simulink model "liftsubsystem"  (R2025b)
settings: Solver=daessc  StartTime=0.0  StopTime=15  FixedStep=1e-3  RelTol=1e-3
values from neighbouring files (symbols this model uses):
  b0 = 1.0    (= 1)    [get_arm_model_with_disturbance.m]    (also in robotParams.m = 3.125)
  beta1 = 3 * omega_o    (= 120)    [robotParams.m]
  beta2 = 3 * omega_o^2    (= 4800)    [robotParams.m]
  beta3 = omega_o^3    (= 64000)    [robotParams.m]
  g = 9.81    [get_arm_model.m]    (also in robotParams.m)
  g_fork = 2*pi*50    (= 314.159265359)    [robotParams.m]
  g_lift = 2*pi*50    (= 314.159265359)    [robotParams.m]
  Kd_fork = 5    [robotParams.m]
  Kd_lift = 5    [robotParams.m]
  Kp_fork = 20    [robotParams.m]
  Kp_lift = 20    [robotParams.m]
  lx = 0.3    [robotParams.m]
  ly = 0.8    [robotParams.m]
  lz = 1    [robotParams.m]
  m = 1    [robotParams.m]
  M = reshape([mt1,mt2,mt3],4,4)    [mass_matrix.m]    (also in robotParams.m = 16)
  m_w = 1    [robotParams.m]
  N = 20    [ocp_arm.m]    (also in ocp_arm_disturbances.m; ocp_lift.m)
  T_control = 1e-3    (= 0.001)    [robotParams.m]
undefined symbols (not defined in the file or in its folder): dspblkCoreblockFVToolHelper, gcbh, K_fd, K_fp, M_n44, Mn_33, Mn_44, X, Y, Z
libraries: sm_lib x257, nesl_utility x58, sharedTrackingLibrary x6, slpidlib x4, simulink x4, robotcorelib x1
(part 1 of 8)
settings Model: Creator=itsan  LastModifiedBy=itsan

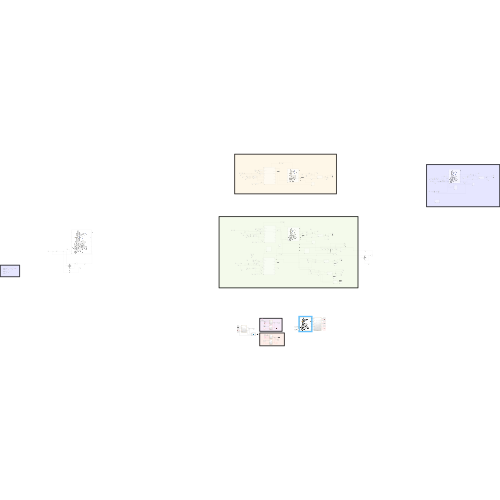
[thumbnail: Simulink's stored preview of the top-level diagram]
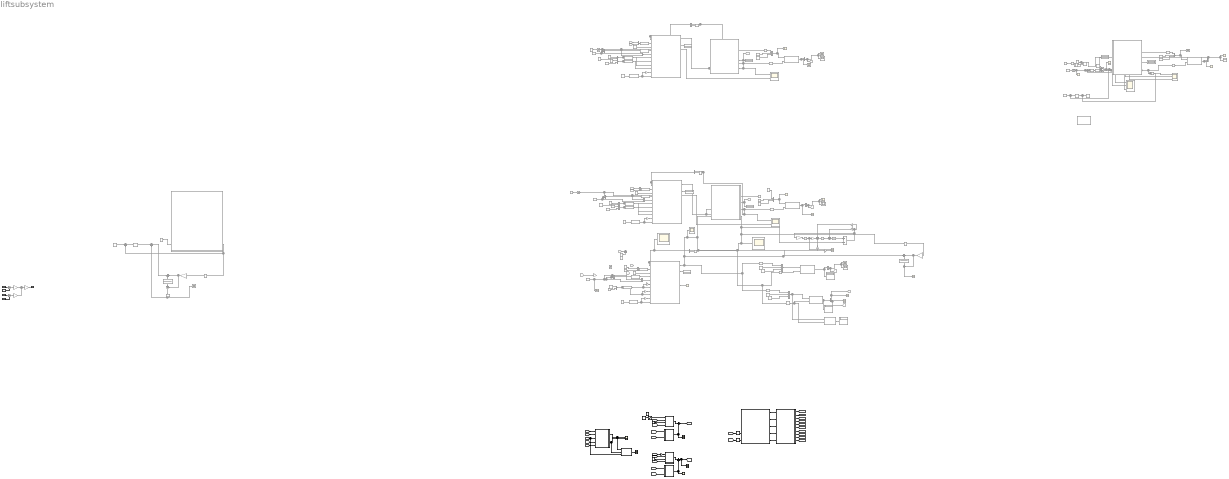
== system liftsubsystem ==
  note: Lift
  Position : Inport
  Velocity : Inport  Port=2
  Position_cmd : Inport  Port=3
  Velocity_cmd : Inport  Port=4
  Calculations : Subsystem
  Constant{,11,16,24..25} (5 alike) : Constant  Commented=on  Value=0.5
  Constant1 : Constant  Commented=on  Value=9.81
  Constant{4,10,15,26,34..35} (6 alike) : Constant  Commented=on  Value=0.01
  Constant12 : Constant  Commented=on  Value=0.8
  Constant{8,13,18,22,30,38} (6 alike) : Constant  Commented=on  Value=0
  Constant14 : Constant  Commented=on  Value=150
  Constant17 : Constant  Commented=on  Value=0.8
  Constant19 : Constant  Commented=on  Value=150
  Constant2 : Constant  Commented=on  Value=12
  Constant20 : Constant  Commented=on  Value=[0 0 0]
  Constant21 : Constant  Commented=on  Value=-0.5
  Constant{3,5,9,23} (4 alike) : Constant  Commented=on  Value=0.43
  Constant27 : Constant  Commented=on  Value=100
  Constant28 : Constant  Commented=on  Value=[0 0 0]
  Constant29 : Constant  Commented=on  Value=7
  Constant31 : Constant  Commented=on  Value=0.4
  Constant{32..33,36..37} (4 alike) : Constant  Commented=on  Value=5
  Constant39 : Constant  Commented=on  Value=-5.99
  Constant42 : Constant  Value=0
  Constant43 : Constant  Value=0
  Constant45 : Constant  Value=0.0
  Constant6 : Constant  Commented=on  Value=[0 0 0]
  Constant7 : Constant  Commented=on  Value=-0.5
  Cos : Trigonometry  Commented=on  Operator=cos
  Delay : Delay  Commented=on
  Demux{,1..3} (4 alike) : Demux  Commented=on  Outputs=3
  Demux4 : Demux  Commented=on
  Derivative{,1..5} (6 alike) : Derivative  Commented=on
  Discrete LPF1 : DiscreteFilter  Commented=on  LoadFcn=dspblkCoreblockFVToolHelper(gcbh,'load');  Numerator=[-5.866*0.001]  Denominator=[1-5.866*0.001 -1]
      settings: CopyFcn=dspblkCoreblockFVToolHelper(gcbh,'copy');  DeleteFcn=dspblkCoreblockFVToolHelper(gcbh,'close');  ModelCloseFcn=dspblkCoreblockFVToolHelper(gcbh,'close');  PreSaveFcn=dspblkCoreblockFVToolHelper(gcbh,'presave');  PostSaveFcn=dspblkCoreblockFVToolHelper(gcbh,'postsave');  CloseFcn=dspblkCoreblockFVToolHelper(gcbh,'close');
  Discrete LPF2 : DiscreteFilter  Commented=on  LoadFcn=dspblkCoreblockFVToolHelper(gcbh,'load');  Numerator=[31*0.001]  Denominator=[1+31*0.001 -1]
      settings: CopyFcn=dspblkCoreblockFVToolHelper(gcbh,'copy');  DeleteFcn=dspblkCoreblockFVToolHelper(gcbh,'close');  ModelCloseFcn=dspblkCoreblockFVToolHelper(gcbh,'close');  PreSaveFcn=dspblkCoreblockFVToolHelper(gcbh,'presave');  PostSaveFcn=dspblkCoreblockFVToolHelper(gcbh,'postsave');  CloseFcn=dspblkCoreblockFVToolHelper(gcbh,'close');
  Display{,1..13} (14 alike) : Display  Commented=on
  Divide : Product  Commented=on  Inputs=***
  Divide1 : Product  Commented=on  Inputs=**
  Extended Kalman Filter : sharedTrackingLibrary/Extended Kalman Filter  Commented=on  StateTransitionFcn=myStateTransitionFcn  HasStateTransitionJacobianFcn=off  HasAdditiveProcessNoise=Additive  ProcessNoise=diag([1e-6, 1e-4, 1e-8])  HasTimeVaryingProcessNoise=off  HasStateTransitionFcnExtraArgument=1  InitialState=[0; 0; 10]  InitialStateCovariance=diag([1e-2, 1e-2, 100])  MeasurementFcn1=myMeasurementFcn  HasMeasurementJacobianFcn1=off  HasMeasurementEnablePort1=off  HasAdditiveMeasurementNoise1=Additive  MeasurementNoise1=diag([1e-2])  HasTimeVaryingMeasurementNoise1=off  HasMeasurementFcnExtraArgument1=0  HasMeasurementWrapping1=off  MeasurementFcn2=myMeasurementFcn  HasMeasurementJacobianFcn2=off  HasMeasurementEnablePort2=off  HasAdditiveMeasurementNoise2=Additive  MeasurementNoise2=1  HasTimeVaryingMeasurementNoise2=off  HasMeasurementFcnExtraArgument2=0  HasMeasurementWrapping2=off  MeasurementFcn3=myMeasurementFcn  HasMeasurementJacobianFcn3=off  HasMeasurementEnablePort3=off  HasAdditiveMeasurementNoise3=Additive  MeasurementNoise3=1  HasTimeVaryingMeasurementNoise3=off  HasMeasurementFcnExtraArgument3=0  HasMeasurementWrapping3=off  MeasurementFcn4=myMeasurementFcn  HasMeasurementJacobianFcn4=off  HasMeasurementEnablePort4=off  HasAdditiveMeasurementNoise4=Additive  MeasurementNoise4=1  HasTimeVaryingMeasurementNoise4=off  HasMeasurementFcnExtraArgument4=0  HasMeasurementWrapping4=off  MeasurementFcn5=myMeasurementFcn  HasMeasurementJacobianFcn5=off  HasMeasurementEnablePort5=off  HasAdditiveMeasurementNoise5=Additive  MeasurementNoise5=1  HasTimeVaryingMeasurementNoise5=off  HasMeasurementFcnExtraArgument5=0  HasMeasurementWrapping5=off  EnableMultirate=off  StateTransitionFcnSampleTime=1  MeasurementFcn1SampleTime=1  MeasurementFcn2SampleTime=1  MeasurementFcn3SampleTime=1  MeasurementFcn4SampleTime=1  MeasurementFcn5SampleTime=1  UseCurrentEstimator=on  OutputStateCovariance=off  DataType=double  SampleTime=0.01  NumberOfMeasurements=1
  Extended Kalman Filter1 : sharedTrackingLibrary/Extended Kalman Filter  Commented=on  StateTransitionFcn=myStateTransitionFcn  HasStateTransitionJacobianFcn=off  HasAdditiveProcessNoise=Additive  ProcessNoise=diag([1e-6, 1e-4, 1e-8])  HasTimeVaryingProcessNoise=off  HasStateTransitionFcnExtraArgument=1  InitialState=[0; 0; 10]  InitialStateCovariance=diag([1e-2, 1e-2, 100])  MeasurementFcn1=myMeasurementFcn  HasMeasurementJacobianFcn1=off  HasMeasurementEnablePort1=off  HasAdditiveMeasurementNoise1=Additive  MeasurementNoise1=diag([1e-2])  HasTimeVaryingMeasurementNoise1=off  HasMeasurementFcnExtraArgument1=0  HasMeasurementWrapping1=off  MeasurementFcn2=myMeasurementFcn  HasMeasurementJacobianFcn2=off  HasMeasurementEnablePort2=off  HasAdditiveMeasurementNoise2=Additive  MeasurementNoise2=1  HasTimeVaryingMeasurementNoise2=off  HasMeasurementFcnExtraArgument2=0  HasMeasurementWrapping2=off  MeasurementFcn3=myMeasurementFcn  HasMeasurementJacobianFcn3=off  HasMeasurementEnablePort3=off  HasAdditiveMeasurementNoise3=Additive  MeasurementNoise3=1  HasTimeVaryingMeasurementNoise3=off  HasMeasurementFcnExtraArgument3=0  HasMeasurementWrapping3=off  MeasurementFcn4=myMeasurementFcn  HasMeasurementJacobianFcn4=off  HasMeasurementEnablePort4=off  HasAdditiveMeasurementNoise4=Additive  MeasurementNoise4=1  HasTimeVaryingMeasurementNoise4=off  HasMeasurementFcnExtraArgument4=0  HasMeasurementWrapping4=off  MeasurementFcn5=myMeasurementFcn  HasMeasurementJacobianFcn5=off  HasMeasurementEnablePort5=off  HasAdditiveMeasurementNoise5=Additive  MeasurementNoise5=1  HasTimeVaryingMeasurementNoise5=off  HasMeasurementFcnExtraArgument5=0  HasMeasurementWrapping5=off  EnableMultirate=off  StateTransitionFcnSampleTime=1  MeasurementFcn1SampleTime=1  MeasurementFcn2SampleTime=1  MeasurementFcn3SampleTime=1  MeasurementFcn4SampleTime=1  MeasurementFcn5SampleTime=1  UseCurrentEstimator=on  OutputStateCovariance=off  DataType=double  SampleTime=0.01  NumberOfMeasurements=1
  Extended Kalman Filter2 : sharedTrackingLibrary/Extended Kalman Filter  Commented=on  StateTransitionFcn=liftStateTransitionFcn  HasStateTransitionJacobianFcn=off  HasAdditiveProcessNoise=Additive  ProcessNoise=diag([1e-6, 1e-4, 1e-8])  HasTimeVaryingProcessNoise=off  HasStateTransitionFcnExtraArgument=1  InitialState=[0; 0; 10]  InitialStateCovariance=diag([1e-2, 1e-2, 100])  MeasurementFcn1=liftMeasurementFcn  HasMeasurementJacobianFcn1=off  HasMeasurementEnablePort1=off  HasAdditiveMeasurementNoise1=Additive  MeasurementNoise1=diag([1e-2])  HasTimeVaryingMeasurementNoise1=off  HasMeasurementFcnExtraArgument1=0  HasMeasurementWrapping1=off  MeasurementFcn2=myMeasurementFcn  HasMeasurementJacobianFcn2=off  HasMeasurementEnablePort2=off  HasAdditiveMeasurementNoise2=Additive  MeasurementNoise2=1  HasTimeVaryingMeasurementNoise2=off  HasMeasurementFcnExtraArgument2=0  HasMeasurementWrapping2=off  MeasurementFcn3=myMeasurementFcn  HasMeasurementJacobianFcn3=off  HasMeasurementEnablePort3=off  HasAdditiveMeasurementNoise3=Additive  MeasurementNoise3=1  HasTimeVaryingMeasurementNoise3=off  HasMeasurementFcnExtraArgument3=0  HasMeasurementWrapping3=off  MeasurementFcn4=myMeasurementFcn  HasMeasurementJacobianFcn4=off  HasMeasurementEnablePort4=off  HasAdditiveMeasurementNoise4=Additive  MeasurementNoise4=1  HasTimeVaryingMeasurementNoise4=off  HasMeasurementFcnExtraArgument4=0  HasMeasurementWrapping4=off  MeasurementFcn5=myMeasurementFcn  HasMeasurementJacobianFcn5=off  HasMeasurementEnablePort5=off  HasAdditiveMeasurementNoise5=Additive  MeasurementNoise5=1  HasTimeVaryingMeasurementNoise5=off  HasMeasurementFcnExtraArgument5=0  HasMeasurementWrapping5=off  EnableMultirate=off  StateTransitionFcnSampleTime=1  MeasurementFcn1SampleTime=1  MeasurementFcn2SampleTime=1  MeasurementFcn3SampleTime=1  MeasurementFcn4SampleTime=1  MeasurementFcn5SampleTime=1  UseCurrentEstimator=on  OutputStateCovariance=off  DataType=double  SampleTime=0.01  NumberOfMeasurements=1
  Extended Kalman Filter3 : sharedTrackingLibrary/Extended Kalman Filter  Commented=on  StateTransitionFcn=armStateTransitionFcn  HasStateTransitionJacobianFcn=off  HasAdditiveProcessNoise=Additive  ProcessNoise=diag([1e-8, 1e-6,1e-10])  HasTimeVaryingProcessNoise=off  HasStateTransitionFcnExtraArgument=1  InitialState=[0;0;0.3]  InitialStateCovariance=diag([1e-4, 1e-4,100])  MeasurementFcn1=armMeasurementFcn  HasMeasurementJacobianFcn1=off  HasMeasurementEnablePort1=off  HasAdditiveMeasurementNoise1=Additive  MeasurementNoise1=1e-4  HasTimeVaryingMeasurementNoise1=off  HasMeasurementFcnExtraArgument1=0  HasMeasurementWrapping1=off  MeasurementFcn2=myMeasurementFcn  HasMeasurementJacobianFcn2=off  HasMeasurementEnablePort2=off  HasAdditiveMeasurementNoise2=Additive  MeasurementNoise2=1  HasTimeVaryingMeasurementNoise2=off  HasMeasurementFcnExtraArgument2=0  HasMeasurementWrapping2=off  MeasurementFcn3=myMeasurementFcn  HasMeasurementJacobianFcn3=off  HasMeasurementEnablePort3=off  HasAdditiveMeasurementNoise3=Additive  MeasurementNoise3=1  HasTimeVaryingMeasurementNoise3=off  HasMeasurementFcnExtraArgument3=0  HasMeasurementWrapping3=off  MeasurementFcn4=myMeasurementFcn  HasMeasurementJacobianFcn4=off  HasMeasurementEnablePort4=off  HasAdditiveMeasurementNoise4=Additive  MeasurementNoise4=1  HasTimeVaryingMeasurementNoise4=off  HasMeasurementFcnExtraArgument4=0  HasMeasurementWrapping4=off  MeasurementFcn5=myMeasurementFcn  HasMeasurementJacobianFcn5=off  HasMeasurementEnablePort5=off  HasAdditiveMeasurementNoise5=Additive  MeasurementNoise5=1  HasTimeVaryingMeasurementNoise5=off  HasMeasurementFcnExtraArgument5=0  HasMeasurementWrapping5=off  EnableMultirate=off  StateTransitionFcnSampleTime=1  MeasurementFcn1SampleTime=1  MeasurementFcn2SampleTime=1  MeasurementFcn3SampleTime=1  MeasurementFcn4SampleTime=1  MeasurementFcn5SampleTime=1  UseCurrentEstimator=on  OutputStateCovariance=off  DataType=double  SampleTime=0.01  NumberOfMeasurements=1
  Extended Kalman Filter5 : sharedTrackingLibrary/Extended Kalman Filter  Commented=on  StateTransitionFcn=armMassStateTransitionFcn  HasStateTransitionJacobianFcn=off  HasAdditiveProcessNoise=Additive  ProcessNoise=diag([1e-8, 1e-6,1e-10,1e-10])  HasTimeVaryingProcessNoise=off  HasStateTransitionFcnExtraArgument=1  InitialState=[0;0;0.3;2]  InitialStateCovariance=diag([1e-4, 1e-4,100,100])  MeasurementFcn1=armMeasurementFcn  HasMeasurementJacobianFcn1=off  HasMeasurementEnablePort1=off  HasAdditiveMeasurementNoise1=Additive  MeasurementNoise1=1e-4  HasTimeVaryingMeasurementNoise1=off  HasMeasurementFcnExtraArgument1=0  HasMeasurementWrapping1=off  MeasurementFcn2=myMeasurementFcn  HasMeasurementJacobianFcn2=off  HasMeasurementEnablePort2=off  HasAdditiveMeasurementNoise2=Additive  MeasurementNoise2=1  HasTimeVaryingMeasurementNoise2=off  HasMeasurementFcnExtraArgument2=0  HasMeasurementWrapping2=off  MeasurementFcn3=myMeasurementFcn  HasMeasurementJacobianFcn3=off  HasMeasurementEnablePort3=off  HasAdditiveMeasurementNoise3=Additive  MeasurementNoise3=1  HasTimeVaryingMeasurementNoise3=off  HasMeasurementFcnExtraArgument3=0  HasMeasurementWrapping3=off  MeasurementFcn4=myMeasurementFcn  HasMeasurementJacobianFcn4=off  HasMeasurementEnablePort4=off  HasAdditiveMeasurementNoise4=Additive  MeasurementNoise4=1  HasTimeVaryingMeasurementNoise4=off  HasMeasurementFcnExtraArgument4=0  HasMeasurementWrapping4=off  MeasurementFcn5=myMeasurementFcn  HasMeasurementJacobianFcn5=off  HasMeasurementEnablePort5=off  HasAdditiveMeasurementNoise5=Additive  MeasurementNoise5=1  HasTimeVaryingMeasurementNoise5=off  HasMeasurementFcnExtraArgument5=0  HasMeasurementWrapping5=off  EnableMultirate=off  StateTransitionFcnSampleTime=1  MeasurementFcn1SampleTime=1  MeasurementFcn2SampleTime=1  MeasurementFcn3SampleTime=1  MeasurementFcn4SampleTime=1  MeasurementFcn5SampleTime=1  UseCurrentEstimator=on  OutputStateCovariance=off  DataType=double  SampleTime=0.01  NumberOfMeasurements=1
  Fork DOB : Subsystem
  From{,2,6..7} (4 alike) : From  Commented=on  GotoTag=Mass
  From1 : From  Commented=on  GotoTag=Pitch
  From3 : From  Commented=on  GotoTag=Pitch
  From4 : From  Commented=on  GotoTag=Pitch
  From5 : From  Commented=on  GotoTag=rx
  Gain{,1..5,12} (7 alike) : Gain  Commented=on  Gain=-1
  Gain10 : Gain  Commented=on  Gain=b0
  Gain11 : Gain  Commented=on  Gain=beta2
  Gain13 : Gain  Commented=on  Gain=beta1
  Gain14 : Gain  Commented=on  Gain=-beta3
  Gain15 : Gain  Commented=on  Gain=b0
  Gain16 : Gain  Commented=on  Gain=31*0.21
  Gain18 : Gain  Gain=-1
  Gain6 : Gain  Commented=on  Gain=K_fp
  Gain7 : Gain  Commented=on  Gain=K_fd
  Gain8 : Gain  Commented=on  Gain=M_n44
  Gain9 : Gain  Commented=on  Gain=-0.21*5.866
  Goto : Goto  Commented=on  GotoTag=Mass
  Goto1 : Goto  Commented=on  GotoTag=Pitch
  Goto2 : Goto  Commented=on  GotoTag=Mass
  Goto3 : Goto  Commented=on  GotoTag=Pitch
  Goto4 : Goto  Commented=on  GotoTag=Mass
  Goto5 : Goto  Commented=on  GotoTag=rx
  Goto6 : Goto  Commented=on  GotoTag=rx
  Lift DOB : Subsystem
  MATLAB Function : MATLAB Function  TreatAsAtomicUnit=on
  Mux{,2,5..8,10,12..15,18..20} (14 alike) : Mux  Commented=on  Inputs=2
  Mux{1,3..4,9,11,16..17,21} (8 alike) : Mux  Commented=on  Inputs=3
  PD : slpidlib/PID Controller  Commented=on  Controller=PID  Form=Parallel  TimeDomain=Continuous-time  UseExternalTs=off  SampleTime=-1  IntegratorMethod=Forward Euler  FilterMethod=Forward Euler  ControllerParametersSource=internal  P=1  I=0.001  UseKiTs=off  D=22  UseExternalDerivativeSource=off  N=15  UseFilter=on  TunerSelectOption=Transfer Function Based (PID Tuner App)  InitialConditionSource=internal  InitialConditionForIntegrator=0  InitialConditionForFilter=0  DifferentiatorICPrevScaledInput=0  ExternalReset=none  TrackingMode=off  Kt=1  LimitOutput=on  SatLimitsSource=internal  UpperSaturationLimit=100  LowerSaturationLimit=-100  LinearizeAsGain=on  AntiWindupMode=back-calculation  Kb=3  LimitIntegrator=off  UpperIntegratorSaturationLimit=inf  LowerIntegratorSaturationLimit=-inf  POutMin=[]  POutMax=[]  IOutMin=[]  IOutMax=[]  DOutMin=[]  DOutMax=[]  NOutMin=[]  NOutMax=[]  SumOutMin=[]  SumOutMax=[]  SaturationOutMin=[]  SaturationOutMax=[]  PParamMin=[]  PParamMax=[]  IParamMin=[]  IParamMax=[]  DParamMin=[]  DParamMax=[]  NParamMin=[]  NParamMax=[]  KbParamMin=[]  KbParamMax=[]  KtParamMin=[]  KtParamMax=[]  KbOutMin=[]  KbOutMax=[]  KtOutMin=[]  KtOutMax=[]  IntegratorOutMin=[]  IntegratorOutMax=[]  FilterOutMin=[]  FilterOutMax=[]  SumI1OutMin=[]  SumI1OutMax=[]  SumI2OutMin=[]  SumI2OutMax=[]  SumI3OutMin=[]  SumI3OutMax=[]  SumI4OutMin=[]  SumI4OutMax=[]  SumDOutMin=[]  SumDOutMax=[]  DifferentiatorOutMin=[]  DifferentiatorOutMax=[]  FilterDiffOutCoefMin=[]  FilterDiffOutCoefMax=[]  ReciprocalOutMin=[]  ReciprocalOutMax=[]  SumDenOutMin=[]  SumDenOutMax=[]  SumNumOutMin=[]  SumNumOutMax=[]  DivideOutMin=[]  DivideOutMax=[]  UdiffTsProdOutMin=[]  UdiffTsProdOutMax=[]  NTsProdOutMin=[]  NTsProdOutMax=[]  UintegralTsProdOutMin=[]  UintegralTsProdOutMax=[]  UngainTsProdOutMin=[]  UngainTsProdOutMax=[]  ClampingZeroOutDataTypeStr=Inherit: Inherit via back propagation  ClampingZeroOutMin=[]  ClampingZeroOutMax=[]  FilterDenConstantOutDataTypeStr=Inherit: Inherit via back propagation  FilterDenConstantOutMin=[]  FilterDenConstantOutMax=[]  PCopyOutDataTypeStr=Inherit: Inherit via back propagation  PCopyOutMin=[]  PCopyOutMax=[]  NCopyOutDataTypeStr=Inherit: Inherit via back propagation  NCopyOutMin=[]  NCopyOutMax=[]  IntegratorContinuousStateAttributes=''  IntegratorStateMustResolveToSignalObject=off  IntegratorRTWStateStorageClass=Auto  FilterContinuousStateAttributes=''  FilterStateMustResolveToSignalObject=off  FilterRTWStateStorageClass=Auto  ParallelPVariant=InternalParameters  IdealPVariant=Disabled  IVariant=InternalParameters  DVariant=InternalParameters  IntegratorVariant=Continuous  SatVariant=Enabled  AWVariant=BackCalculation  PCopyVariant=Disabled  TRVariant=Disabled  FdbkBlocksVariant=Forward  IdealPFdbkVariant=Disabled  SatFdbkVariant=Disabled  DerivativeFilterVariant=ContFilter  NVariant=InternalParameters  NCopyVariant=Disabled  FilterICVariant=InternalICsFilter  IntegratorICVariant=InternalICs  ExternalResetVariant=Disabled  TRSumVariant=Passthrough  SumFdbkVariant=Disabled  SumVariant=Sum_PID  TsampFilterVariant=InternalTs  TsampNgainVariant=Passthrough  TsampIntegralVariant=Disabled_SignalSpec  ExternalSaturationOutDataTypeStr=Inherit: Same as second input  DerivativeSourceVariant=ErrorSignal  PreIntVariant=InternalPreInt
  PD fork : Subsystem
  PD lift : Subsystem
  PID Controller : slpidlib/PID Controller  Commented=on  Controller=PID  Form=Parallel  TimeDomain=Continuous-time  UseExternalTs=off  SampleTime=-1  IntegratorMethod=Forward Euler  FilterMethod=Forward Euler  ControllerParametersSource=internal  P=10  I=0  UseKiTs=off  D=0  UseExternalDerivativeSource=off  N=0  UseFilter=on  TunerSelectOption=Transfer Function Based (PID Tuner App)  InitialConditionSource=internal  InitialConditionForIntegrator=0  InitialConditionForFilter=0  DifferentiatorICPrevScaledInput=0  ExternalReset=none  TrackingMode=off  Kt=1  LimitOutput=on  SatLimitsSource=internal  UpperSaturationLimit=1  LowerSaturationLimit=-1  LinearizeAsGain=on  AntiWindupMode=none  Kb=1  LimitIntegrator=off  UpperIntegratorSaturationLimit=inf  LowerIntegratorSaturationLimit=-inf  POutMin=[]  POutMax=[]  IOutMin=[]  IOutMax=[]  DOutMin=[]  DOutMax=[]  NOutMin=[]  NOutMax=[]  SumOutMin=[]  SumOutMax=[]  SaturationOutMin=[]  SaturationOutMax=[]  PParamMin=[]  PParamMax=[]  IParamMin=[]  IParamMax=[]  DParamMin=[]  DParamMax=[]  NParamMin=[]  NParamMax=[]  KbParamMin=[]  KbParamMax=[]  KtParamMin=[]  KtParamMax=[]  KbOutMin=[]  KbOutMax=[]  KtOutMin=[]  KtOutMax=[]  IntegratorOutMin=[]  IntegratorOutMax=[]  FilterOutMin=[]  FilterOutMax=[]  SumI1OutMin=[]  SumI1OutMax=[]  SumI2OutMin=[]  SumI2OutMax=[]  SumI3OutMin=[]  SumI3OutMax=[]  SumI4OutMin=[]  SumI4OutMax=[]  SumDOutMin=[]  SumDOutMax=[]  DifferentiatorOutMin=[]  DifferentiatorOutMax=[]  FilterDiffOutCoefMin=[]  FilterDiffOutCoefMax=[]  ReciprocalOutMin=[]  ReciprocalOutMax=[]  SumDenOutMin=[]  SumDenOutMax=[]  SumNumOutMin=[]  SumNumOutMax=[]  DivideOutMin=[]  DivideOutMax=[]  UdiffTsProdOutMin=[]  UdiffTsProdOutMax=[]  NTsProdOutMin=[]  NTsProdOutMax=[]  UintegralTsProdOutMin=[]  UintegralTsProdOutMax=[]  UngainTsProdOutMin=[]  UngainTsProdOutMax=[]  ClampingZeroOutDataTypeStr=Inherit: Inherit via back propagation  ClampingZeroOutMin=[]  ClampingZeroOutMax=[]  FilterDenConstantOutDataTypeStr=Inherit: Inherit via back propagation  FilterDenConstantOutMin=[]  FilterDenConstantOutMax=[]  PCopyOutDataTypeStr=Inherit: Inherit via back propagation  PCopyOutMin=[]  PCopyOutMax=[]  NCopyOutDataTypeStr=Inherit: Inherit via back propagation  NCopyOutMin=[]  NCopyOutMax=[]  IntegratorContinuousStateAttributes=''  IntegratorStateMustResolveToSignalObject=off  IntegratorRTWStateStorageClass=Auto  FilterContinuousStateAttributes=''  FilterStateMustResolveToSignalObject=off  FilterRTWStateStorageClass=Auto  ParallelPVariant=InternalParameters  IdealPVariant=Disabled  IVariant=InternalParameters  DVariant=InternalParameters  IntegratorVariant=Continuous  SatVariant=Enabled  AWVariant=Passthrough  PCopyVariant=Disabled  TRVariant=Disabled  FdbkBlocksVariant=Forward  IdealPFdbkVariant=Disabled  SatFdbkVariant=Disabled  DerivativeFilterVariant=ContFilter  NVariant=InternalParameters  NCopyVariant=Disabled  FilterICVariant=InternalICsFilter  IntegratorICVariant=InternalICs  ExternalResetVariant=Disabled  TRSumVariant=Passthrough  SumFdbkVariant=Disabled  SumVariant=Sum_PID  TsampFilterVariant=InternalTs  TsampNgainVariant=Passthrough  TsampIntegralVariant=Disabled_SignalSpec  ExternalSaturationOutDataTypeStr=Inherit: Same as second input  DerivativeSourceVariant=ErrorSignal  PreIntVariant=InternalPreInt
  PID Controller1 : slpidlib/PID Controller  Commented=on  Controller=PID  Form=Parallel  TimeDomain=Continuous-time  UseExternalTs=off  SampleTime=-1  IntegratorMethod=Forward Euler  FilterMethod=Forward Euler  ControllerParametersSource=internal  P=10  I=4  UseKiTs=off  D=0  UseExternalDerivativeSource=off  N=0  UseFilter=on  TunerSelectOption=Transfer Function Based (PID Tuner App)  InitialConditionSource=internal  InitialConditionForIntegrator=0  InitialConditionForFilter=0  DifferentiatorICPrevScaledInput=0  ExternalReset=none  TrackingMode=off  Kt=1  LimitOutput=on  SatLimitsSource=internal  UpperSaturationLimit=1  LowerSaturationLimit=-1  LinearizeAsGain=on  AntiWindupMode=none  Kb=1  LimitIntegrator=off  UpperIntegratorSaturationLimit=inf  LowerIntegratorSaturationLimit=-inf  POutMin=[]  POutMax=[]  IOutMin=[]  IOutMax=[]  DOutMin=[]  DOutMax=[]  NOutMin=[]  NOutMax=[]  SumOutMin=[]  SumOutMax=[]  SaturationOutMin=[]  SaturationOutMax=[]  PParamMin=[]  PParamMax=[]  IParamMin=[]  IParamMax=[]  DParamMin=[]  DParamMax=[]  NParamMin=[]  NParamMax=[]  KbParamMin=[]  KbParamMax=[]  KtParamMin=[]  KtParamMax=[]  KbOutMin=[]  KbOutMax=[]  KtOutMin=[]  KtOutMax=[]  IntegratorOutMin=[]  IntegratorOutMax=[]  FilterOutMin=[]  FilterOutMax=[]  SumI1OutMin=[]  SumI1OutMax=[]  SumI2OutMin=[]  SumI2OutMax=[]  SumI3OutMin=[]  SumI3OutMax=[]  SumI4OutMin=[]  SumI4OutMax=[]  SumDOutMin=[]  SumDOutMax=[]  DifferentiatorOutMin=[]  DifferentiatorOutMax=[]  FilterDiffOutCoefMin=[]  FilterDiffOutCoefMax=[]  ReciprocalOutMin=[]  ReciprocalOutMax=[]  SumDenOutMin=[]  SumDenOutMax=[]  SumNumOutMin=[]  SumNumOutMax=[]  DivideOutMin=[]  DivideOutMax=[]  UdiffTsProdOutMin=[]  UdiffTsProdOutMax=[]  NTsProdOutMin=[]  NTsProdOutMax=[]  UintegralTsProdOutMin=[]  UintegralTsProdOutMax=[]  UngainTsProdOutMin=[]  UngainTsProdOutMax=[]  ClampingZeroOutDataTypeStr=Inherit: Inherit via back propagation  ClampingZeroOutMin=[]  ClampingZeroOutMax=[]  FilterDenConstantOutDataTypeStr=Inherit: Inherit via back propagation  FilterDenConstantOutMin=[]  FilterDenConstantOutMax=[]  PCopyOutDataTypeStr=Inherit: Inherit via back propagation  PCopyOutMin=[]  PCopyOutMax=[]  NCopyOutDataTypeStr=Inherit: Inherit via back propagation  NCopyOutMin=[]  NCopyOutMax=[]  IntegratorContinuousStateAttributes=''  IntegratorStateMustResolveToSignalObject=off  IntegratorRTWStateStorageClass=Auto  FilterContinuousStateAttributes=''  FilterStateMustResolveToSignalObject=off  FilterRTWStateStorageClass=Auto  ParallelPVariant=InternalParameters  IdealPVariant=Disabled  IVariant=InternalParameters  DVariant=InternalParameters  IntegratorVariant=Continuous  SatVariant=Enabled  AWVariant=Passthrough  PCopyVariant=Disabled  TRVariant=Disabled  FdbkBlocksVariant=Forward  IdealPFdbkVariant=Disabled  SatFdbkVariant=Disabled  DerivativeFilterVariant=ContFilter  NVariant=InternalParameters  NCopyVariant=Disabled  FilterICVariant=InternalICsFilter  IntegratorICVariant=InternalICs  ExternalResetVariant=Disabled  TRSumVariant=Passthrough  SumFdbkVariant=Disabled  SumVariant=Sum_PID  TsampFilterVariant=InternalTs  TsampNgainVariant=Passthrough  TsampIntegralVariant=Disabled_SignalSpec  ExternalSaturationOutDataTypeStr=Inherit: Same as second input  DerivativeSourceVariant=ErrorSignal  PreIntVariant=InternalPreInt
  PID Controller2 : slpidlib/PID Controller  Commented=on  Controller=PID  Form=Parallel  TimeDomain=Continuous-time  UseExternalTs=off  SampleTime=-1  IntegratorMethod=Forward Euler  FilterMethod=Forward Euler  ControllerParametersSource=internal  P=1  I=0  UseKiTs=off  D=1  UseExternalDerivativeSource=off  N=100  UseFilter=on  TunerSelectOption=Transfer Function Based (PID Tuner App)  InitialConditionSource=internal  InitialConditionForIntegrator=0  InitialConditionForFilter=0  DifferentiatorICPrevScaledInput=0  ExternalReset=none  TrackingMode=off  Kt=1  LimitOutput=off  SatLimitsSource=internal  UpperSaturationLimit=inf  LowerSaturationLimit=-inf  LinearizeAsGain=on  AntiWindupMode=none  Kb=1  LimitIntegrator=off  UpperIntegratorSaturationLimit=inf  LowerIntegratorSaturationLimit=-inf  POutMin=[]  POutMax=[]  IOutMin=[]  IOutMax=[]  DOutMin=[]  DOutMax=[]  NOutMin=[]  NOutMax=[]  SumOutMin=[]  SumOutMax=[]  SaturationOutMin=[]  SaturationOutMax=[]  PParamMin=[]  PParamMax=[]  IParamMin=[]  IParamMax=[]  DParamMin=[]  DParamMax=[]  NParamMin=[]  NParamMax=[]  KbParamMin=[]  KbParamMax=[]  KtParamMin=[]  KtParamMax=[]  KbOutMin=[]  KbOutMax=[]  KtOutMin=[]  KtOutMax=[]  IntegratorOutMin=[]  IntegratorOutMax=[]  FilterOutMin=[]  FilterOutMax=[]  SumI1OutMin=[]  SumI1OutMax=[]  SumI2OutMin=[]  SumI2OutMax=[]  SumI3OutMin=[]  SumI3OutMax=[]  SumI4OutMin=[]  SumI4OutMax=[]  SumDOutMin=[]  SumDOutMax=[]  DifferentiatorOutMin=[]  DifferentiatorOutMax=[]  FilterDiffOutCoefMin=[]  FilterDiffOutCoefMax=[]  ReciprocalOutMin=[]  ReciprocalOutMax=[]  SumDenOutMin=[]  SumDenOutMax=[]  SumNumOutMin=[]  SumNumOutMax=[]  DivideOutMin=[]  DivideOutMax=[]  UdiffTsProdOutMin=[]  UdiffTsProdOutMax=[]  NTsProdOutMin=[]  NTsProdOutMax=[]  UintegralTsProdOutMin=[]  UintegralTsProdOutMax=[]  UngainTsProdOutMin=[]  UngainTsProdOutMax=[]  ClampingZeroOutDataTypeStr=Inherit: Inherit via back propagation  ClampingZeroOutMin=[]  ClampingZeroOutMax=[]  FilterDenConstantOutDataTypeStr=Inherit: Inherit via back propagation  FilterDenConstantOutMin=[]  FilterDenConstantOutMax=[]  PCopyOutDataTypeStr=Inherit: Inherit via back propagation  PCopyOutMin=[]  PCopyOutMax=[]  NCopyOutDataTypeStr=Inherit: Inherit via back propagation  NCopyOutMin=[]  NCopyOutMax=[]  IntegratorContinuousStateAttributes=''  IntegratorStateMustResolveToSignalObject=off  IntegratorRTWStateStorageClass=Auto  FilterContinuousStateAttributes=''  FilterStateMustResolveToSignalObject=off  FilterRTWStateStorageClass=Auto  ParallelPVariant=InternalParameters  IdealPVariant=Disabled  IVariant=InternalParameters  DVariant=InternalParameters  IntegratorVariant=Continuous  SatVariant=Disabled  AWVariant=Passthrough  PCopyVariant=Disabled  TRVariant=Disabled  FdbkBlocksVariant=Forward  IdealPFdbkVariant=Disabled  SatFdbkVariant=Disabled  DerivativeFilterVariant=ContFilter  NVariant=InternalParameters  NCopyVariant=Disabled  FilterICVariant=InternalICsFilter  IntegratorICVariant=InternalICs  ExternalResetVariant=Disabled  TRSumVariant=Passthrough  SumFdbkVariant=Disabled  SumVariant=Sum_PID  TsampFilterVariant=InternalTs  TsampNgainVariant=Passthrough  TsampIntegralVariant=Disabled_SignalSpec  ExternalSaturationOutDataTypeStr=Inherit: Same as second input  DerivativeSourceVariant=ErrorSignal  PreIntVariant=InternalPreInt
  Plant1 : Subsystem  Commented=on
      mask Display: image('plant.png');
  Plant2 : Subsystem  Commented=on
      mask Display: image('plant.png');
  Plant3 : Subsystem  Commented=on
      mask Display: image('plant.png');
  Plant4 : Subsystem  Commented=on
      mask Display: image('plant.png');
  Plant5 : Subsystem
      mask Display: image('plant.png');
  Ramp : simulink/Sources/Ramp  Commented=on  slope=0.5  start=0  InitialOutput=0
  Ramp1 : simulink/Sources/Ramp  Commented=on  slope=1  start=0  InitialOutput=0
  Ramp2 : simulink/Sources/Ramp  slope=0.05  start=1  InitialOutput=0
  Ramp3 : simulink/Sources/Ramp  Commented=on  slope=1  start=0  InitialOutput=0
  Rate Transition : RateTransition  OutPortSampleTime=T_control
  Rate Transition1 : RateTransition  OutPortSampleTime=T_control
  S-Function : S-Function  Commented=on  FunctionName=repmat_sfun  Parameters=N+1  SFunctionDeploymentMode=off  EnableBusSupport=off
  S-Function1 : S-Function  Commented=on  FunctionName=acados_solver_sfunction_linear_actuator_model  SFunctionDeploymentMode=off  EnableBusSupport=off
      mask Display:
      | % from the make_sfun file
      | global sfun_input_names sfun_output_names
      | for i = 1:length(sfun_input_names)
      | 	port_label('input', i, sfun_input_names{i})
      | end
      | for i = 1:length(sfun_output_names)
      | 	port_label('output', i, sfun_output_names{i})
      | end
  S-Function{2..4,8..10,12,16} (8 alike) : S-Function  Commented=on  FunctionName=repmat_sfun  Parameters=N-1  SFunctionDeploymentMode=off  EnableBusSupport=off
  S-Function11 : S-Function  Commented=on  FunctionName=repmat_sfun  Parameters=N  SFunctionDeploymentMode=off  EnableBusSupport=off
  S-Function13 : S-Function  Commented=on  FunctionName=repmat_sfun  Parameters=N  SFunctionDeploymentMode=off  EnableBusSupport=off
  S-Function14 : S-Function  Commented=on  FunctionName=repmat_sfun  Parameters=N+1  SFunctionDeploymentMode=off  EnableBusSupport=off
  S-Function15 : S-Function  Commented=on  FunctionName=acados_solver_sfunction_arm_model  SFunctionDeploymentMode=off  EnableBusSupport=off
      mask Display:
      | % from the make_sfun file
      | global sfun_input_names sfun_output_names
      | for i = 1:length(sfun_input_names)
      | 	port_label('input', i, sfun_input_names{i})
      | end
      | for i = 1:length(sfun_output_names)
      | 	port_label('output', i, sfun_output_names{i})
      | end
  S-Function5 : S-Function  Commented=on  FunctionName=repmat_sfun  Parameters=N  SFunctionDeploymentMode=off  EnableBusSupport=off
  S-Function6 : S-Function  Commented=on  FunctionName=repmat_sfun  Parameters=N+1  SFunctionDeploymentMode=off  EnableBusSupport=off
  S-Function7 : S-Function  Commented=on  FunctionName=acados_solver_sfunction_linear_actuator_model  SFunctionDeploymentMode=off  EnableBusSupport=off
      mask Display:
      | % from the make_sfun file
      | global sfun_input_names sfun_output_names
      | for i = 1:length(sfun_input_names)
      | 	port_label('input', i, sfun_input_names{i})
      | end
      | for i = 1:length(sfun_output_names)
      | 	port_label('output', i, sfun_output_names{i})
      | end
  Saturation : Saturate  Commented=on
  Saturation1 : Saturate  Commented=on
  Saturation2 : Saturate  UpperLimit=.25
  Saturation3 : Saturate  Commented=on  UpperLimit=0.1
  Scope{,2..4,6,8..11,13..23,25} (21 alike) : Scope  Commented=on
      Scope settings: ActiveDisplayYMinimum=117.38726606594429  ActiveDisplayYMaximum=117.96497291719386
      Scope10 settings: ActiveDisplayYMinimum=10.368033685081326  ActiveDisplayYMaximum=13.754521835601309  DataLoggingVariableName=ScopeData7
      Scope11 settings: ActiveDisplayYMinimum=-23.500486572497707  ActiveDisplayYMaximum=44.300288166456191  DataLoggingVariableName=ScopeData9
      Scope13 settings: ActiveDisplayYMinimum=-23.500486572497707  ActiveDisplayYMaximum=44.300288166456191  DataLoggingVariableName=ScopeData10
      Scope14 settings: ActiveDisplayYMinimum=-23.500486572497707  ActiveDisplayYMaximum=44.300288166456191  DataLoggingVariableName=ScopeData12
      Scope15 settings: ActiveDisplayYMinimum=-1  ActiveDisplayYMaximum=1  DataLoggingVariableName=ScopeData21
      Scope16 settings: ActiveDisplayYMinimum=-0.065967569407599264  ActiveDisplayYMaximum=0.0325873905390409  DataLoggingVariableName=ScopeData22
      Scope17 settings: ActiveDisplayYMinimum=-12.264920720176846  ActiveDisplayYMaximum=-8.5595612380933073  DataLoggingVariableName=ScopeData23
      Scope18 settings: ActiveDisplayYMinimum=-0.06438015181759206  ActiveDisplayYMaximum=0.57942136635832864  DataLoggingVariableName=ScopeData24
      Scope19 settings: ActiveDisplayYMinimum=-2.6074541865236367  ActiveDisplayYMaximum=1.3784984258302824  DataLoggingVariableName=ScopeData25
      Scope2 settings: ActiveDisplayYMinimum=-23.500486572497707  ActiveDisplayYMaximum=44.300288166456191  DataLoggingVariableName=ScopeData2
      Scope20 settings: ActiveDisplayYMinimum=-0.38236324419750722  ActiveDisplayYMaximum=1.1874760943553313  DataLoggingVariableName=ScopeData26
      Scope21 settings: ActiveDisplayYMinimum=-1.9405440716154967  ActiveDisplayYMaximum=6.5730775878456438  DataLoggingVariableName=ScopeData27
      Scope22 settings: ActiveDisplayYMinimum=-44.337351995967424  ActiveDisplayYMaximum=305.78581856249957  DataLoggingVariableName=ScopeData28
      Scope23 settings: ActiveDisplayYMinimum=-1  ActiveDisplayYMaximum=1  DataLoggingVariableName=ScopeData29
      Scope25 settings: ActiveDisplayYMinimum=-17.016489579172408  ActiveDisplayYMaximum=-16.711425975731455  DataLoggingVariableName=ScopeData31
      Scope3 settings: ActiveDisplayYMinimum=9.4746445379021456  ActiveDisplayYMaximum=14.728199158880699  DataLoggingVariableName=ScopeData3
      Scope4 settings: ActiveDisplayYMinimum=-0.93767561156709411  ActiveDisplayYMaximum=3.3247649685442195  DataLoggingVariableName=ScopeData4
      Scope6 settings: ActiveDisplayYMinimum=-23.500486572497707  ActiveDisplayYMaximum=44.300288166456191  DataLoggingVariableName=ScopeData6
      Scope8 settings: ActiveDisplayYMinimum=1.7628570115484123  ActiveDisplayYMaximum=12.261814228718583  DataLoggingVariableName=ScopeData19
      Scope9 settings: ActiveDisplayYMinimum=-23.500486572497707  ActiveDisplayYMaximum=44.300288166456191  DataLoggingVariableName=ScopeData13
  Scope1 : Scope  Commented=on  NumInputPorts=3
      settings: ActiveDisplayYMinimum=-0.20308839711342824  ActiveDisplayYMaximum=1.2259812299014095
  Scope12 : Scope  Commented=on  NumInputPorts=2
      settings: ActiveDisplayYMinimum=-0.12609078655591466  ActiveDisplayYMaximum=0.56374645055007666  DataLoggingVariableName=ScopeData11
  Scope24 : Scope  Commented=on  NumInputPorts=2
      settings: ActiveDisplayYMinimum=16.110993442444876  ActiveDisplayYMaximum=19.010475082855386  DataLoggingVariableName=ScopeData30
  Scope26 : Scope  NumInputPorts=2
      settings: ActiveDisplayYMinimum=-10.259307517283297  ActiveDisplayYMaximum=12.749109094986899  DataLoggingVariableName=ScopeData32
  Scope{27,29..31} (4 alike) : Scope
      Scope27 settings: ActiveDisplayYMinimum=0.72040252232650048  ActiveDisplayYMaximum=1.0503294124696438  DataLoggingVariableName=ScopeData33
      Scope29 settings: ActiveDisplayYMinimum=-84.4164918961249  ActiveDisplayYMaximum=78.859392305860567  DataLoggingVariableName=ScopeData36
      Scope30 settings: ActiveDisplayYMinimum=-31.694740506194762  ActiveDisplayYMaximum=285.25266455575292  DataLoggingVariableName=ScopeData35
      Scope31 settings: ActiveDisplayYMinimum=-80.561540487267592  ActiveDisplayYMaximum=-19.024576924749461  DataLoggingVariableName=ScopeData37
  Scope5 : Scope  Commented=on  NumInputPorts=3
      settings: ActiveDisplayYMinimum=-3.3927367175447758  ActiveDisplayYMaximum=3.8241131199467557  DataLoggingVariableName=ScopeData5
  Scope7 : Scope  Commented=on  NumInputPorts=2
      settings: ActiveDisplayYMinimum=-0.12609078655591466  ActiveDisplayYMaximum=0.56374645055007666  DataLoggingVariableName=ScopeData8
  Signal Specification : SignalSpecification  Commented=on  OutDataTypeStr=double  Dimensions=1
  Step : Step  Commented=on  Time=2  Before=2  After=3  SampleTime=0
  Subsystem : Subsystem
  Subtract : Sum  Commented=on  Inputs=+-
  Sum{,2..4,6..7,10,15} (8 alike) : Sum  Commented=on  Inputs=|+-
  Sum1 : Sum  Commented=on  Inputs=+|+
  Sum11 : Sum  Commented=on  Inputs=|++
  Sum12 : Sum  Commented=on  Inputs=-+|
  Sum13 : Sum  Commented=on  Inputs=-++
  Sum14 : Sum  Commented=on  Inputs=+|+
  Sum16 : Sum  Inputs=|++
  Sum17 : Sum  Inputs=|++
  Sum5 : Sum  Commented=on  Inputs=|++
  Sum8 : Sum  Commented=on  Inputs=|++
  Sum9 : Sum  Commented=on  Inputs=+|+
  Trapezoidal Velocity Profile Trajectory : robotcorelib/Trapezoidal Velocity Profile Trajectory  Commented=on  WaypointSource=Internal  Waypoints=[ 0, -0.5, -1; 0, 0.5, 1 ]  NumParams=0  Parameter1=Peak Velocity  Parameter2=End Time  ParameterSource=Internal  PeakVelocity=[ 2; 2 ]  Acceleration=[ 1; 2 ]  EndTime=[ 1; 1 ]  AccelTime=[ 1; 2 ]  SimulateUsing=Code generation
  Unscented Kalman Filter1 : sharedTrackingLibrary/Unscented Kalman Filter  Commented=on  StateTransitionFcn=armMassStateTransitionUKF  HasAdditiveProcessNoise=Additive  ProcessNoise=diag([1e-8, 1e-6,1e-3])  HasTimeVaryingProcessNoise=off  HasStateTransitionFcnExtraArgument=1  InitialState=[0;0;0.5]  InitialStateCovariance=diag([1e-4, 1e-3, 0.2])  Alpha=1e-3  Beta=2  Kappa=0  MeasurementFcn1=armMeasurementUKF  HasMeasurementEnablePort1=off  HasAdditiveMeasurementNoise1=Additive  MeasurementNoise1=1e-4  HasTimeVaryingMeasurementNoise1=off  HasMeasurementFcnExtraArgument1=0  HasMeasurementWrapping1=off  MeasurementFcn2=myMeasurementFcn  HasMeasurementEnablePort2=off  HasAdditiveMeasurementNoise2=Additive  MeasurementNoise2=1  HasTimeVaryingMeasurementNoise2=off  HasMeasurementFcnExtraArgument2=0  HasMeasurementWrapping2=off  MeasurementFcn3=myMeasurementFcn  HasMeasurementEnablePort3=off  HasAdditiveMeasurementNoise3=Additive  MeasurementNoise3=1  HasTimeVaryingMeasurementNoise3=off  HasMeasurementFcnExtraArgument3=0  HasMeasurementWrapping3=off  MeasurementFcn4=myMeasurementFcn  HasMeasurementEnablePort4=off  HasAdditiveMeasurementNoise4=Additive  MeasurementNoise4=1  HasTimeVaryingMeasurementNoise4=off  HasMeasurementFcnExtraArgument4=0  HasMeasurementWrapping4=off  MeasurementFcn5=myMeasurementFcn  HasMeasurementEnablePort5=off  HasAdditiveMeasurementNoise5=Additive  MeasurementNoise5=1  HasTimeVaryingMeasurementNoise5=off  HasMeasurementFcnExtraArgument5=0  HasMeasurementWrapping5=off  EnableMultirate=off  StateTransitionFcnSampleTime=1  MeasurementFcn1SampleTime=1  MeasurementFcn2SampleTime=1  MeasurementFcn3SampleTime=1  MeasurementFcn4SampleTime=1  MeasurementFcn5SampleTime=1  UseCurrentEstimator=on  OutputStateCovariance=off  DataType=double  SampleTime=0.01  NumberOfMeasurements=1
      settings: LibrarySourceBlock=cstblocks/State Estimation/Unscented Kalman Filter
  Zero-Order Hold{,1..9} (10 alike) : ZeroOrderHold  Commented=on  SampleTime=0.01
  int1 : Integrator  Commented=on
  int2 : Integrator  Commented=on
  int3 : Integrator  Commented=on
  Torque_ref : Outport
  wires:
  Sum/1 -> PID Controller/1
  Constant/1 -> Sum/1
  Constant1/1 -> Divide1/2, Divide/1
  Derivative/1 -> Sum2/2
  PID Controller/1 -> Sum2/1
  Sum2/1 -> PID Controller1/1
  Extended Kalman Filter/1 -> Scope2/1, Demux/1
  Plant1/4(lift_pos) -> Sum3/2, Sum/2, Scope5/3, Zero-Order Hold2/1, Derivative/1, Scope1/1
  Demux/3 -> Scope3/1, Display/1, Divide1/1
  Saturation/1 -> Scope1/2, Sum3/1, Scope4/1  "ref"
  Constant4/1 -> Mux3/2
  Sum1/1 -> Scope/1, Scope5/1, Zero-Order Hold1/1, Plant1/4(liftForce), Display2/1  "utotal"
  Signal Specification/1 -> Scope5/2, Sum1/2  "upid"
  Ramp/1 -> Saturation/1
  PD/1 -> Signal Specification/1
  Sum3/1 -> Scope1/3, PD/1  "error"
  Constant3/1 -> Mux3/3
  Zero-Order Hold1/1 -> Mux3/1
  Zero-Order Hold2/1 -> Extended Kalman Filter/2
  Mux3/1 -> Extended Kalman Filter/1, Scope6/1  "inputs"
  Constant2/1 -> Divide/3
  Cos/1 -> Divide/2
  Plant1/3(pitch_angle) -> Display1/1  "pitch_angle"
  Constant5/1 -> Cos/1
  Divide1/1 -> Sum1/1
  Constant10/1 -> Mux1/2
  Plant2/4(lift_pos) -> Scope7/1, Zero-Order Hold4/1, Derivative1/1, Mux/1
  Extended Kalman Filter1/1 -> Scope9/1, Demux1/1
  Mux1/1 -> Extended Kalman Filter1/1, Scope13/1  "inputs"
  Zero-Order Hold4/1 -> Extended Kalman Filter1/2
  Demux1/3 -> Goto/1, Scope10/1, Display3/1
  Zero-Order Hold3/1 -> Mux1/1
  Plant2/3(pitch_angle) -> Goto1/1, Display4/1  "pitch_angle"
  Constant9/1 -> Mux1/3
  Derivative1/1 -> Mux/2
  Mux/1 -> S-Function1/2, S-Function1/1
  S-Function1/1 -> Zero-Order Hold3/1, Plant2/4(liftForce)  "u"
  S-Function1/2 -> Display5/1
  Constant6/1 -> S-Function1/4
  S-Function/1 -> S-Function1/3
  Mux2/1 -> S-Function/1
  S-Function2/1 -> S-Function1/5
  Ramp1/1 -> Saturation1/1
  Saturation1/1 -> Mux7/1, Scope7/2, Mux4/1
  Constant8/1 -> Mux7/2, Mux4/3, Mux4/2
  Mux4/1 -> S-Function2/1
  S-Function3/1 -> S-Function1/7
  Constant7/1 -> Mux5/2
  Mux5/1 -> S-Function1/9, S-Function3/1
  S-Function4/1 -> S-Function1/8
  Constant12/1 -> Mux6/1
  Constant11/1 -> Mux6/2
  Mux6/1 -> S-Function1/10, S-Function4/1
  Constant13/1 -> Mux5/1
  Gain/1 -> S-Function1/11
  S-Function5/1 -> Gain/1, S-Function1/12
  Constant14/1 -> S-Function5/1
  Mux7/1 -> S-Function1/6
  From/1 -> Mux2/1
  From1/1 -> Mux2/2
  From2/1 -> Mux10/1
  Extended Kalman Filter2/1 -> Scope14/1, Demux2/1
  S-Function7/1 -> Zero-Order Hold5/1, Plant3/4(liftForce)  "u"
  Constant22/1 -> Mux14/2, Mux11/3, Mux11/2
  Constant19/1 -> S-Function11/1
  Mux13/1 -> S-Function7/10, S-Function10/1
  S-Function7/2 -> Display8/1
  Mux11/1 -> S-Function8/1
  S-Function9/1 -> S-Function7/7
  Constant23/1 -> Mux9/3
  Demux2/3 -> Goto2/1, Scope8/1, Display6/1
  S-Function8/1 -> S-Function7/5
  Mux12/1 -> S-Function7/9, S-Function9/1
  Constant15/1 -> Mux9/2
  Constant18/1 -> Mux12/1
  From3/1 -> Mux10/2
  Constant20/1 -> S-Function7/4
  Constant16/1 -> Mux13/2
  S-Function11/1 -> Gain1/1, S-Function7/12
  Mux14/1 -> S-Function7/6
  Constant21/1 -> Mux12/2
  Plant3/4(lift_pos) -> Scope12/1, Zero-Order Hold6/1, Mux8/1, Derivative2/1
  Mux8/1 -> S-Function7/2, S-Function7/1
  Mux9/1 -> Extended Kalman Filter2/1, Scope11/1  "inputs"
  Mux10/1 -> S-Function6/1
  Constant17/1 -> Mux13/1
  S-Function6/1 -> S-Function7/3
  Zero-Order Hold6/1 -> Extended Kalman Filter2/2
  S-Function10/1 -> S-Function7/8
  Plant3/3(pitch_angle) -> Display7/1, Goto3/1  "pitch_angle"
  Derivative2/1 -> Mux8/2
  Saturation3/1 -> Mux11/1, Mux14/1, Scope12/2
  Gain1/1 -> S-Function7/11
  Gain2/1 -> S-Function15/11
  Mux15/1 -> S-Function14/1
  Constant25/1 -> Mux18/1
  S-Function14/1 -> S-Function15/3
  S-Function12/1 -> Gain3/1, S-Function15/8
  Mux19/1 -> S-Function15/6
  Constant24/1 -> Mux18/2
  Constant28/1 -> S-Function15/4
  S-Function16/1 -> S-Function15/5
  Constant27/1 -> S-Function13/1
  Mux18/1 -> Gain4/1, S-Function15/10, S-Function12/1
  S-Function15/2 -> Display9/1
  Gain3/1 -> S-Function15/7
  Mux16/1 -> S-Function16/1
  S-Function13/1 -> Gain2/1, S-Function15/12
  Mux20/1 -> S-Function15/2, S-Function15/1, Scope18/1
  Derivative3/1 -> Mux20/2
  Gain4/1 -> S-Function15/9
  Constant26/1 -> Mux9/1
  From4/1 -> Gain5/1
  Zero-Order Hold/1 -> Extended Kalman Filter3/2
  Mux17/1 -> Extended Kalman Filter3/1
  Zero-Order Hold7/1 -> Mux17/1
  Constant33/1 -> Mux17/2
  Constant34/1 -> Mux17/3
  Demux3/3 -> Goto6/1, Display10/1, Scope19/1
  Extended Kalman Filter3/1 -> Demux3/1, Display13/1
  Constant30/1 -> Mux19/2, Mux16/3, Mux16/2, Mux19/1, Mux16/1, Scope15/1
  S-Function15/1 -> Sum14/1, Gain12/1, Plant3/5(armTorque), Gain15/1, Scope17/1, Zero-Order Hold9/1, Zero-Order Hold7/1  "u"
  Extended Kalman Filter5/1 -> Demux4/1, Display11/1
  Mux21/1 -> Unscented Kalman Filter1/1, Extended Kalman Filter5/1
  Constant32/1 -> Mux21/2
  Constant35/1 -> Mux21/3
  Zero-Order Hold9/1 -> Mux21/1
  Demux4/3 -> Goto5/1, Scope20/1
  Demux4/4 -> Goto4/1, Scope21/1
  Ramp3/1 -> Saturation3/1
  From6/1 -> Sum4/1
  Constant29/1 -> Sum4/2
  Unscented Kalman Filter1/1 -> Display12/1
  Zero-Order Hold8/1 -> Unscented Kalman Filter1/2, Extended Kalman Filter5/2
  Sum5/1 -> PID Controller2/1
  Constant38/1 -> Sum5/1
  Gain7/1 -> Sum8/2
  Position/1 -> Sum6/2
  Velocity/1 -> Sum7/2
  Sum8/1 -> Gain8/1
  Sum7/1 -> Gain7/1
  Sum6/1 -> Gain6/1  "Fork error"
  Gain6/1 -> Sum8/1
  Velocity_cmd/1 -> Sum7/1
  Gain8/1 -> Torque_ref/1
  Position_cmd/1 -> Sum6/1
  Gain9/1 -> Sum9/2, Sum10/2
  Sum9/1 -> Discrete LPF1/1
  Delay/1 -> Scope22/1, Sum11/2
  Sum10/1 -> Delay/1
  Derivative4/1 -> Gain9/1
  Sum11/1 -> Sum9/1
  Discrete LPF1/1 -> Sum10/1
  Plant4/5(armPos) -> Sum5/2, Derivative4/1
  PID Controller2/1 -> Sum11/1
  Constant39/1 -> Plant4/5(armTorque)
  Constant31/1 -> Mux15/2
  S-Function15/4 -> Scope23/1
  Plant3/5(armPos) -> Derivative5/1, Scope16/1, Derivative3/1, Mux20/1, Zero-Order Hold8/1, Zero-Order Hold/1, Subtract/2
  int1/1 -> Subtract/1
  Subtract/1 -> Gain11/1, Gain13/1, Gain14/1  "error"
  Sum12/1 -> int1/1  "e"
  int2/1 -> Sum12/2
  Gain13/1 -> Sum12/1
  Sum13/1 -> int2/1  "e"
  int3/1 -> Scope24/1, Gain10/1  "dist"
  Gain11/1 -> Sum13/1
  Gain15/1 -> Sum13/3
  Gain14/1 -> int3/1
  Gain10/1 -> Sum13/2
  Constant36/1 -> Mux15/1
  Gain12/1 -> Scope24/2
  Discrete LPF2/1 -> Sum15/1
  Derivative5/1 -> Gain16/1
  Sum14/1 -> Discrete LPF2/1
  Sum15/1 -> Scope25/1
  Gain16/1 -> Sum15/2, Sum14/2
  Plant5/5(armPos) -> Calculations/5(arm_angle)
  Gain18/1 -> PD fork/1(posRef)
  Plant5/1(rw_angle) -> Calculations/1(rw_angle)  "rw_angle"
  Plant5/2(lw_angle) -> Calculations/2(lw_angle)  "lw_angle"
  Plant5/3(pitch_angle) -> Calculations/3(pitch_angle)  "pitch_angle"
  Plant5/4(lift_pos) -> Calculations/4(lift_height)
  Calculations/1(rw_pos) -> [rw_pos]
  Calculations/2(rw_vel) -> [rw_vel]
  Calculations/3(lw_pos) -> [lw_pos]
  Calculations/4(lw_vel) -> [lw_vel]
  Calculations/10(arm_vel) -> [arm_vel]
  Calculations/9(arm_pos) -> [arm_pos]
  Calculations/8(lift_vel) -> [lift_vel]
  Calculations/7(lift_pos) -> [lift_pos]
  Calculations/6(pitch_vel) -> [pitch_vel]
  Calculations/5(pitch_pos) -> [pitch_pos]
  PD fork/1(out) -> Sum16/1
  Fork DOB/1(Est_dis) -> Scope29/1, Sum16/2
  [arm_pos] -> PD fork/2(posMeas)
  [arm_vel] -> Fork DOB/2(Velocity)
  Sum16/1 -> Scope31/1, [torque_arm]
  [torque_arm] -> Fork DOB/1(Input Torque)
  [torque_arm] -> Rate Transition/1
  [force_lift] -> Rate Transition1/1
  Constant42/1 -> PD fork/3(velRef)
  [arm_vel] -> PD fork/4(velMeas)
  Rate Transition/1 -> Plant5/5(armTorque)
  Rate Transition1/1 -> Plant5/4(liftForce)
  [lift_vel] -> PD lift/4(velMeas)
  Constant43/1 -> PD lift/3(velRef)
  [force_lift] -> Lift DOB/1(Input Torque)
  Sum17/1 -> [force_lift]
  [lift_vel] -> Lift DOB/2(Velocity)
  [lift_pos] -> PD lift/2(posMeas)
  Lift DOB/1(Est_dis) -> Sum17/2, Scope30/1
  PD lift/1(out) -> Sum17/1
  Ramp2/1 -> Saturation2/1
  [pitch_pos] -> Gain18/1
  Saturation2/1 -> PD lift/1(posRef)
  [force_lift] -> Subsystem/1(force_lift)
  [pitch_pos] -> Subsystem/2(pitch_pos)
  [arm_pos] -> Subsystem/4(arm_pos)
  [torque_arm] -> Subsystem/5(torque_arm)
  [lift_pos] -> MATLAB Function/3(height), Subsystem/3(lift_pos)
  Subsystem/1(mass_hat) -> MATLAB Function/1(mass), Scope26/1
  Subsystem/2(dist_hat) -> MATLAB Function/2(distance), Scope26/2
  MATLAB Function/1(cog_new) -> Scope27/1

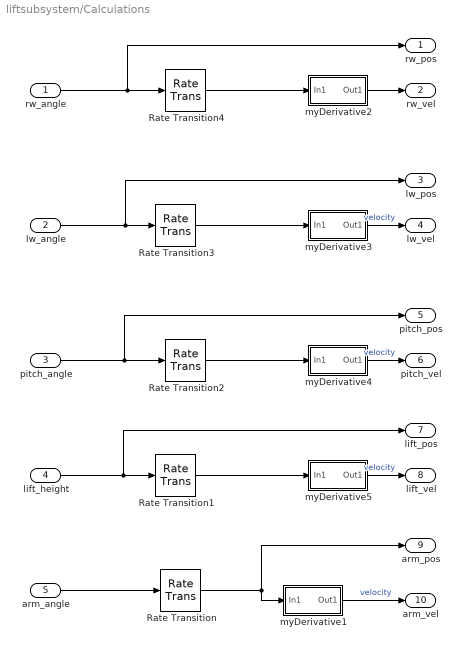
== system liftsubsystem/Calculations ==
  rw_angle : Inport
  lw_angle : Inport  Port=2
  pitch_angle : Inport  Port=3
  lift_height : Inport  Port=4
  arm_angle : Inport  Port=5
  Rate Transition{,1..4} (5 alike) : RateTransition  OutPortSampleTime=T_control
  myDerivative1 : Subsystem
      mask Display: image('myDerivative.png');
  myDerivative2 : Subsystem
      mask Display: image('myDerivative.png');
  myDerivative3 : Subsystem
      mask Display: image('myDerivative.png');
  myDerivative4 : Subsystem
      mask Display: image('myDerivative.png');
  myDerivative5 : Subsystem
      mask Display: image('myDerivative.png');
  rw_pos : Outport
  rw_vel : Outport  Port=2
  lw_pos : Outport  Port=3
  lw_vel : Outport  Port=4
  pitch_pos : Outport  Port=5
  pitch_vel : Outport  Port=6
  lift_pos : Outport  Port=7
  lift_vel : Outport  Port=8
  arm_pos : Outport  Port=9
  arm_vel : Outport  Port=10
  wires:
  Rate Transition4/1 -> myDerivative2/1(In1)
  rw_angle/1 -> Rate Transition4/1, rw_pos/1
  lw_angle/1 -> Rate Transition3/1, lw_pos/1
  Rate Transition3/1 -> myDerivative3/1(In1)
  Rate Transition2/1 -> myDerivative4/1(In1)
  pitch_angle/1 -> Rate Transition2/1, pitch_pos/1
  Rate Transition1/1 -> myDerivative5/1(In1)
  myDerivative2/1(Out1) -> rw_vel/1
  myDerivative3/1(Out1) -> lw_vel/1  "velocity"
  myDerivative4/1(Out1) -> pitch_vel/1  "velocity"
  myDerivative5/1(Out1) -> lift_vel/1  "velocity"
  lift_height/1 -> Rate Transition1/1, lift_pos/1
  arm_angle/1 -> Rate Transition/1
  myDerivative1/1(Out1) -> arm_vel/1  "velocity"
  Rate Transition/1 -> arm_pos/1, myDerivative1/1(In1)
